simulink model "Model_Controlled_2019b"  (R2019b)
settings: Solver=VariableStepAuto  StartTime=0.0  StopTime=0.3  RelTol=1e-3
values from neighbouring files (symbols this model uses):
  Controller1 = kp1*(s*tz+1)*(s*ti+1)/(s*ti*(s*tp+1))    [IntegrationProject.m]
  Controller2 = kp2*(s*tz+1)*(s*ti+1)/(s*ti*(s*tp+1))    [IntegrationProject.m]
  F1 = G1.Denominator{1}(3)/(G1.Numerator{1}(3))    [IntegrationProject.m]
  F2 = G2.Denominator{1}(5)/(G2.Numerator{1}(5))    [IntegrationProject.m]
  G1 = sys_dec(1,1)    [IntegrationProject.m]
  G2 = sys_dec(2,2)    [IntegrationProject.m]
settings Model: Creator=Víctor Carmona  LastModifiedBy=Víctor Carmona
settings DataIOCC: ReturnWorkspaceOutputs=off

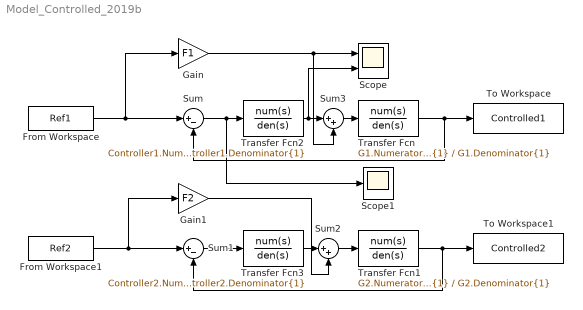
== system Model_Controlled_2019b ==
  From Workspace : FromWorkspace  VariableName=Ref1  SampleTime=2e-4
  From Workspace1 : FromWorkspace  VariableName=Ref2  SampleTime=2e-4
  Gain : Gain  Gain=F1
  Gain1 : Gain  Gain=F2
  Scope : Scope  NumInputPorts=2
  Scope1 : Scope
  Sum : Sum  Inputs=|+-
  Sum1 : Sum  Inputs=|+-
  Sum2 : Sum  Inputs=|++
  Sum3 : Sum  Inputs=|++
  To Workspace : ToWorkspace  VariableName=Controlled1  SaveFormat=Timeseries  SampleTime=-1
  To Workspace1 : ToWorkspace  VariableName=Controlled2  SaveFormat=Timeseries  SampleTime=-1
  Transfer Fcn : TransferFcn  Numerator=G1.Numerator{1}  Denominator=G1.Denominator{1}
  Transfer Fcn1 : TransferFcn  Numerator=G2.Numerator{1}  Denominator=G2.Denominator{1}
  Transfer Fcn2 : TransferFcn  Numerator=Controller1.Numerator{1}  Denominator=Controller1.Denominator{1}
  Transfer Fcn3 : TransferFcn  Numerator=Controller2.Numerator{1}  Denominator=Controller2.Denominator{1}
  wires:
  Transfer Fcn1/1 -> To Workspace1/1, Sum1/2
  From Workspace/1 -> Gain/1, Sum/1
  Sum/1 -> Scope1/1, Transfer Fcn2/1
  Sum1/1 -> Transfer Fcn3/1
  From Workspace1/1 -> Gain1/1, Sum1/1
  Transfer Fcn/1 -> To Workspace/1, Sum/2
  Transfer Fcn3/1 -> Sum2/1
  Sum2/1 -> Transfer Fcn1/1
  Gain1/1 -> Sum2/2
  Transfer Fcn2/1 -> Scope/2, Sum3/1
  Sum3/1 -> Transfer Fcn/1
  Gain/1 -> Sum3/2, Scope/1
